simulink model "Quadrotor_Inner_Loop"  (Simulink 7.6)
settings: Solver=FixedStepDiscrete  StartTime=0.0  StopTime=10.0  FixedStep=0.01  RelTol=1e-3
libraries: passive_control x1
CloseFcn:
  | rtwprivate ssgencode ModelCloseRequest Quadrotor_Inner_Loop
settings Model: Creator=jporter  LastModifiedBy=Administrator
settings DataIOCC: LimitDataPoints=off  SaveOutput=off  SignalLogging=off  DSMLogging=off  SaveTime=off
settings OptimizationCC: InlineParams=on  EnhancedBackFolding=on  PassReuseOutputArgsAs=Individual arguments  OptimizeModelRefInitCode=on
settings HardwareCC: ProdLargestAtomicInteger=Long  ProdLargestAtomicFloat=Float  ProdIntDivRoundTo=Floor  ProdEndianess=LittleEndian  ProdHWDeviceType=ARM Compatible->ARM 7  TargetLargestAtomicInteger=Long  TargetLargestAtomicFloat=Float  TargetIntDivRoundTo=Floor  TargetEndianess=LittleEndian  TargetHWDeviceType=ARM Compatible->ARM 7
settings RTWCC: SystemTargetFile=ert.tlc  GenCodeOnly=on  TemplateMakefile=ert_default_tmf  Description=Real-Time Workshop Embedded Coder  GenerateReport=on  ProcessScript=ert_make_rtw_hook  IncludeHyperlinkInReport=on  LaunchReport=on  GenerateTraceReportSl=on  GenerateTraceReportEml=on  RTWCompilerOptimization=On  CheckMdlBeforeBuild=Warning
settings CodeAppCC: IgnoreCustomStorageClasses=off
settings ERTTargetCC: MultiwordLength=2048  GenerateSampleERTMain=on  CombineSignalStateStructs=on  MultiInstanceERTCode=on  SupportComplex=off  MultiInstanceErrorCode=Warning  ERTCustomFileTemplate=example_file_process.tlc

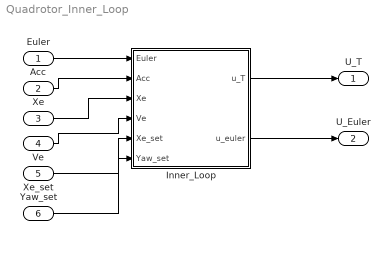
== system Quadrotor_Inner_Loop ==
  Euler : Inport  OutDataTypeStr=single  PortDimensions=[3]
  Acc : Inport  Port=2  OutDataTypeStr=single  PortDimensions=[3]
  Xe : Inport  Port=3  OutDataTypeStr=single  PortDimensions=[3]
  Ve : Inport  Port=4  OutDataTypeStr=single  PortDimensions=[3]
  Xe_set : Inport  Port=5  OutDataTypeStr=single  PortDimensions=[3]
  Yaw_set : Inport  Port=6  OutDataTypeStr=single  PortDimensions=[1]
  Inner_Loop : Subsystem
  U_T : Outport
  U_Euler : Outport  Port=2
  wires:
  Euler/1 -> Inner_Loop/1(Euler)
  Acc/1 -> Inner_Loop/2(Acc)
  Xe/1 -> Inner_Loop/3(Xe)
  Inner_Loop/1(u_T) -> U_T/1
  Inner_Loop/2(u_euler) -> U_Euler/1
  Ve/1 -> Inner_Loop/4(Ve)
  Xe_set/1 -> Inner_Loop/5(Xe_set)
  Yaw_set/1 -> Inner_Loop/6(Yaw_set)

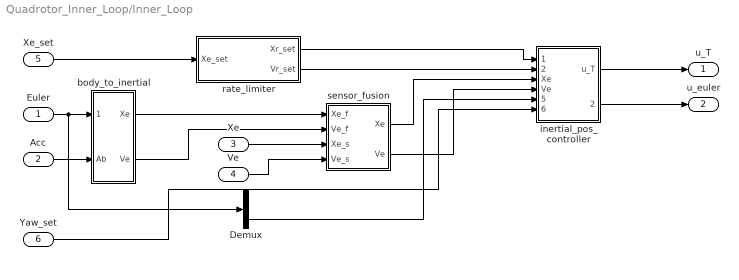
== system Quadrotor_Inner_Loop/Inner_Loop ==
  Euler : Inport  OutDataTypeStr=single  PortDimensions=[3]
  Acc : Inport  Port=2  OutDataTypeStr=single  PortDimensions=[3]
  Xe : Inport  Port=3  OutDataTypeStr=single  PortDimensions=[3]
  Ve : Inport  Port=4  OutDataTypeStr=single  PortDimensions=[3]
  Xe_set : Inport  Port=5  OutDataTypeStr=single  PortDimensions=[3]
  Yaw_set : Inport  Port=6  OutDataTypeStr=single  PortDimensions=[1]
  Demux : Demux  Outputs=3
  body_to_inertial : Subsystem
  inertial_pos_controller : Subsystem
  rate_limiter : Subsystem  mask{wn=2*pi, zeta=0.9, Vmax=2, Ts=0.01}
      mask prompts: wn "omega_n"; Vmax "Max velocity"; Ts "Sample time"
      mask init:
      | Hs_v=tf([2*zeta*wn],[1,2*zeta*wn]);
      | Hz_v=ipesh_transform(Hs_v,Ts);
      | Hs_i=tf([1],[1,0]);
      | Hz_i=ipesh_transform(Hs_i,Ts);
  sensor_fusion : Subsystem  mask{tau=.1, Ts=.01, Ts_gps=.1}
      mask prompts: tau "low-pass time constant (sec) [tau]"; Ts "Sample time [Ts]"; Ts_gps "GPS Sample Time [Ts_gps]"
  u_T : Outport  OutDataTypeStr=single  PortDimensions=[1]
  u_euler : Outport  Port=2  OutDataTypeStr=single  PortDimensions=[3]
  wires:
  Xe_set/1 -> rate_limiter/1(Xe_set)
  inertial_pos_controller/2(u_euler) -> u_euler/1
  Euler/1 -> body_to_inertial/1(euler), Demux/1
  Acc/1 -> body_to_inertial/2(Ab)
  sensor_fusion/1(Xe) -> inertial_pos_controller/3(Xe)
  sensor_fusion/2(Ve) -> inertial_pos_controller/4(Ve)
  body_to_inertial/1(Xe) -> sensor_fusion/1(Xe_f)
  body_to_inertial/2(Ve) -> sensor_fusion/2(Ve_f)
  Xe/1 -> sensor_fusion/3(Xe_s)
  Ve/1 -> sensor_fusion/4(Ve_s)
  rate_limiter/1(Xr_set) -> inertial_pos_controller/1(Xe_set)
  Demux/3 -> inertial_pos_controller/5(Yaw_actual)
  Yaw_set/1 -> inertial_pos_controller/6(Yaw_set)
  rate_limiter/2(Vr_set) -> inertial_pos_controller/2(Ve_set)
  inertial_pos_controller/1(u_T) -> u_T/1

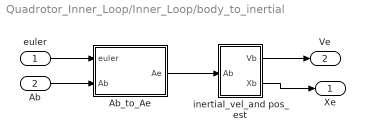
== system Quadrotor_Inner_Loop/Inner_Loop/body_to_inertial ==
  euler : Inport
  Ab : Inport  Port=2
  Ab_to_Ae : Stateflow chart  TreatAsAtomicUnit=on
  inertial_vel_and pos_est : Subsystem  mask{Ts=.01}
      mask prompts: Ts "Sample Time [Ts] (seconds):"
  Xe : Outport
  Ve : Outport  Port=2
  wires:
  euler/1 -> Ab_to_Ae/1(euler)
  Ab/1 -> Ab_to_Ae/2(Ab)
  Ab_to_Ae/1(Ae) -> inertial_vel_and pos_est/1(Ab)
  inertial_vel_and pos_est/1(Vb) -> Ve/1
  inertial_vel_and pos_est/2(Xb) -> Xe/1

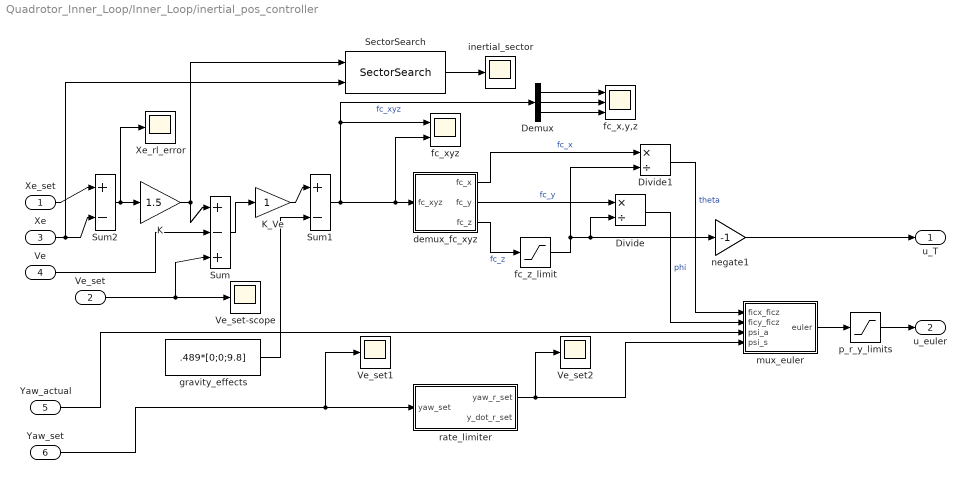
== system Quadrotor_Inner_Loop/Inner_Loop/inertial_pos_controller ==
  Xe_set : Inport
  Ve_set : Inport  Port=2
  Xe : Inport  Port=3
  Ve : Inport  Port=4
  Yaw_actual : Inport  Port=5
  Yaw_set : Inport  Port=6
  Demux : Demux  Outputs=3
  Divide : Product  Inputs=*/  OutDataTypeStr=single
  Divide1 : Product  Inputs=*/  OutDataTypeStr=single
  K : Gain  Gain=1.5  OutDataTypeStr=single
  K_Ve : Gain  ParamDataTypeStr=single  OutDataTypeStr=single
  SectorSearch : passive_control/SectorSearch  SystemSampleTime=-1
  Sum : Sum  Inputs=|+-+  AccumDataTypeStr=single  OutDataTypeStr=single
  Sum1 : Sum  Inputs=|+-  AccumDataTypeStr=single  OutDataTypeStr=single
  Sum2 : Sum  Inputs=|+-  AccumDataTypeStr=single  OutDataTypeStr=single
  Ve_set-scope : Scope
      settings: TimeRange=60  YMin=-2  YMax=2  SaveName=ScopeData2  Decimation=10
  Ve_set1 : Scope
      settings: TimeRange=60  YMin=-1  YMax=1  SaveName=ScopeData10  Decimation=10
  Ve_set2 : Scope
      settings: TimeRange=60  YMin=-1  YMax=1  SaveName=ScopeData11  Decimation=10
  Xe_rl_error : Scope
      settings: TimeRange=80  YMin=-1  YMax=1  SaveName=inertial_sector_data1  MaxDataPoints=50000
  demux_fc_xyz : Stateflow chart  TreatAsAtomicUnit=on
  fc_x,y,z : Scope  NumInputPorts=3
      settings: TimeRange=80  YMin=-1~-5~-5  YMax=1~5~5  SaveName=inertial_sector_data3  MaxDataPoints=50000
  fc_xyz : Scope  NumInputPorts=2
      settings: TimeRange=80  YMin=-1~-5  YMax=1~5  SaveName=inertial_sector_data2  MaxDataPoints=50000
  fc_z_limit : Saturate  UpperLimit=-(1/8)*3.7  LowerLimit=-4*3.7  OutDataTypeStr=single
  gravity_effects : Constant  Value=.489*[0;0;9.8]  OutDataTypeStr=single  SampleTime=.01
  inertial_sector : Scope
      settings: TimeRange=80  YMin=-1  YMax=1  SaveName=inertial_sector_data  MaxDataPoints=50000
  mux_euler : Stateflow chart  TreatAsAtomicUnit=on
  negate1 : Gain  Gain=-1  OutDataTypeStr=single
  p_r_y_limits : Saturate  UpperLimit=[pi/4,pi/4,inf]  LowerLimit=-[pi/4,pi/4,inf]  OutDataTypeStr=single
  rate_limiter : Subsystem  mask{wn=1, zeta=0.9, Vmax=2, Ts=0.01}
      mask prompts: wn "omega_n"; Vmax "Max velocity"; Ts "Sample time"
      mask init:
      | Hs_v=tf([2*zeta*wn],[1,2*zeta*wn]);
      | Hz_v=ipesh_transform(Hs_v,Ts);
      | Hs_i=tf([1],[1,0]);
      | Hz_i=ipesh_transform(Hs_i,Ts);
  u_T : Outport
  u_euler : Outport  Port=2
  wires:
  fc_z_limit/1 -> Divide1/2, Divide/2, negate1/1
  Xe_set/1 -> Sum2/1
  negate1/1 -> u_T/1
  p_r_y_limits/1 -> u_euler/1
  demux_fc_xyz/1(fc_x) -> Divide1/1  "fc_x"
  demux_fc_xyz/3(fc_z) -> fc_z_limit/1  "fc_z"
  mux_euler/1(euler) -> p_r_y_limits/1
  gravity_effects/1 -> Sum1/2
  Sum/1 -> K_Ve/1
  Xe/1 -> Sum2/2, SectorSearch/2
  Sum2/1 -> K/1, Xe_rl_error/1
  demux_fc_xyz/2(fc_y) -> Divide/1  "fc_y"
  K_Ve/1 -> Sum1/1
  Ve/1 -> Sum/2
  Divide1/1 -> mux_euler/1(ficx_ficz)  "theta"
  Divide/1 -> mux_euler/2(ficy_ficz)  "phi"
  Yaw_set/1 -> Ve_set1/1, rate_limiter/1(yaw_set)
  Yaw_actual/1 -> mux_euler/3(psi_a)
  SectorSearch/1 -> inertial_sector/1
  K/1 -> Sum/1, SectorSearch/1
  Ve_set/1 -> Sum/3, Ve_set-scope/1
  Sum1/1 -> fc_xyz/1, Demux/1, demux_fc_xyz/1(fc_xyz), fc_xyz/2  "fc_xyz"
  rate_limiter/1(yaw_r_set) -> mux_euler/4(psi_s), Ve_set2/1
  Demux/1 -> fc_x,y,z/1
  Demux/2 -> fc_x,y,z/2
  Demux/3 -> fc_x,y,z/3

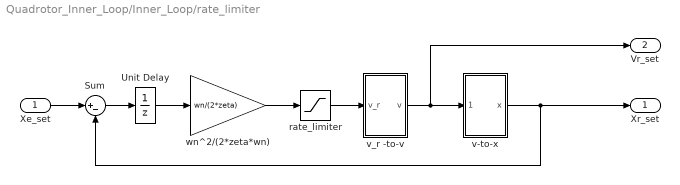
== system Quadrotor_Inner_Loop/Inner_Loop/rate_limiter ==
  Xe_set : Inport
  Sum : Sum  Inputs=|+-
  Unit Delay : UnitDelay  SampleTime=-1
  rate_limiter : Saturate  UpperLimit=Vmax*[1,1,1]  LowerLimit=-Vmax*[1,1,1]
  v-to-x : Subsystem
  v_r -to-v : Subsystem
  wn^2/(2*zeta*wn) : Gain  Gain=wn/(2*zeta)
  Xr_set : Outport
  Vr_set : Outport  Port=2
  wires:
  v_r -to-v/1(v) -> v-to-x/1(x_dot), Vr_set/1
  v-to-x/1(x) -> Sum/2, Xr_set/1
  rate_limiter/1 -> v_r -to-v/1(v_r)
  Xe_set/1 -> Sum/1
  Sum/1 -> Unit Delay/1
  wn^2/(2*zeta*wn)/1 -> rate_limiter/1
  Unit Delay/1 -> wn^2/(2*zeta*wn)/1

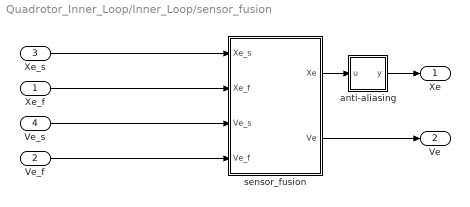
== system Quadrotor_Inner_Loop/Inner_Loop/sensor_fusion ==
  Xe_f : Inport
  Ve_f : Inport  Port=2
  Xe_s : Inport  Port=3
  Ve_s : Inport  Port=4
  anti-aliasing : Subsystem  mask{tau=tau, Ts=Ts}
      mask prompts: tau "tau (sec)"; Ts "Ts (sec)"
      mask init:
      | Hs = tf(1,[tau,1]);
      | Hz = ipesh_transform(Hs,Ts);
  sensor_fusion : Stateflow chart  TreatAsAtomicUnit=on
  Xe : Outport
  Ve : Outport  Port=2
  wires:
  Xe_f/1 -> sensor_fusion/2(Xe_f)
  Ve_f/1 -> sensor_fusion/4(Ve_f)
  sensor_fusion/1(Xe) -> anti-aliasing/1(u)
  anti-aliasing/1(y) -> Xe/1
  Xe_s/1 -> sensor_fusion/1(Xe_s)
  sensor_fusion/2(Ve) -> Ve/1
  Ve_s/1 -> sensor_fusion/3(Ve_s)

== system Quadrotor_Inner_Loop/Inner_Loop/body_to_inertial/inertial_vel_and pos_est ==
  Ab : Inport
  DT_integrator : Subsystem
  DT_integrator1 : Subsystem
  Vb : Outport
  Xb : Outport  Port=2
  wires:
  DT_integrator1/1(Xb) -> Xb/1
  Ab/1 -> DT_integrator/1(Ab)
  DT_integrator/1(Vb) -> Vb/1, DT_integrator1/1(Vb)

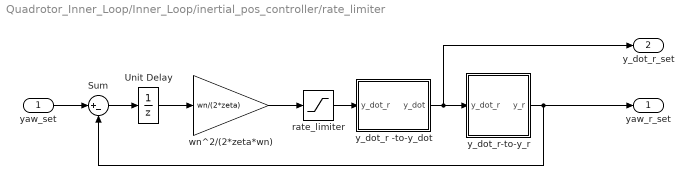
== system Quadrotor_Inner_Loop/Inner_Loop/inertial_pos_controller/rate_limiter ==
  yaw_set : Inport
  Sum : Sum  Inputs=|+-
  Unit Delay : UnitDelay  SampleTime=-1
  rate_limiter : Saturate  UpperLimit=Vmax  LowerLimit=-Vmax
  wn^2/(2*zeta*wn) : Gain  Gain=wn/(2*zeta)
  y_dot_r -to-y_dot : Subsystem
  y_dot_r-to-y_r : Subsystem
  yaw_r_set : Outport
  y_dot_r_set : Outport  Port=2
  wires:
  Unit Delay/1 -> wn^2/(2*zeta*wn)/1
  wn^2/(2*zeta*wn)/1 -> rate_limiter/1
  Sum/1 -> Unit Delay/1
  yaw_set/1 -> Sum/1
  rate_limiter/1 -> y_dot_r -to-y_dot/1(y_dot_r)
  y_dot_r-to-y_r/1(y_r) -> yaw_r_set/1, Sum/2
  y_dot_r -to-y_dot/1(y_dot) -> y_dot_r_set/1, y_dot_r-to-y_r/1(y_dot_r)

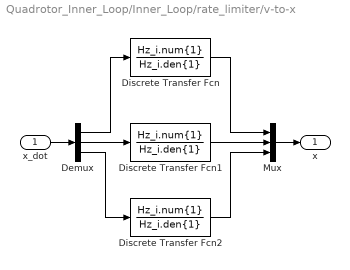
== system Quadrotor_Inner_Loop/Inner_Loop/rate_limiter/v-to-x ==
  x_dot : Inport
  Demux : Demux  Outputs=3
  Discrete Transfer Fcn : DiscreteTransferFcn  Numerator=Hz_i.num{1}  Denominator=Hz_i.den{1}  SampleTime=-1
  Discrete Transfer Fcn1 : DiscreteTransferFcn  Numerator=Hz_i.num{1}  Denominator=Hz_i.den{1}  SampleTime=-1
  Discrete Transfer Fcn2 : DiscreteTransferFcn  Numerator=Hz_i.num{1}  Denominator=Hz_i.den{1}  SampleTime=-1
  Mux : Mux  Inputs=3
  x : Outport
  wires:
  Mux/1 -> x/1
  x_dot/1 -> Demux/1
  Discrete Transfer Fcn2/1 -> Mux/3
  Demux/3 -> Discrete Transfer Fcn2/1
  Discrete Transfer Fcn1/1 -> Mux/2
  Demux/2 -> Discrete Transfer Fcn1/1
  Discrete Transfer Fcn/1 -> Mux/1
  Demux/1 -> Discrete Transfer Fcn/1

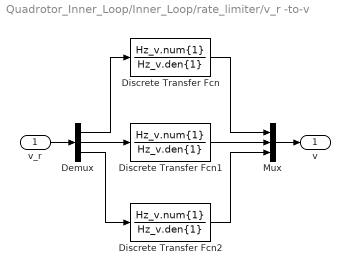
== system Quadrotor_Inner_Loop/Inner_Loop/rate_limiter/v_r -to-v ==
  v_r : Inport
  Demux : Demux  Outputs=3
  Discrete Transfer Fcn : DiscreteTransferFcn  Numerator=Hz_v.num{1}  Denominator=Hz_v.den{1}  SampleTime=-1
  Discrete Transfer Fcn1 : DiscreteTransferFcn  Numerator=Hz_v.num{1}  Denominator=Hz_v.den{1}  SampleTime=-1
  Discrete Transfer Fcn2 : DiscreteTransferFcn  Numerator=Hz_v.num{1}  Denominator=Hz_v.den{1}  SampleTime=-1
  Mux : Mux  Inputs=3
  v : Outport
  wires:
  Demux/1 -> Discrete Transfer Fcn/1
  Discrete Transfer Fcn/1 -> Mux/1
  Demux/2 -> Discrete Transfer Fcn1/1
  Discrete Transfer Fcn1/1 -> Mux/2
  Demux/3 -> Discrete Transfer Fcn2/1
  Discrete Transfer Fcn2/1 -> Mux/3
  v_r/1 -> Demux/1
  Mux/1 -> v/1

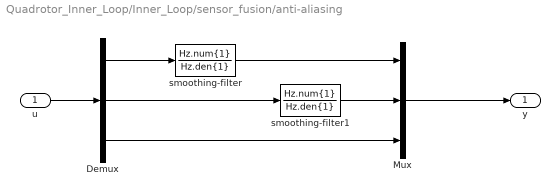
== system Quadrotor_Inner_Loop/Inner_Loop/sensor_fusion/anti-aliasing ==
  u : Inport
  Demux : Demux  Outputs=3
  Mux : Mux  Inputs=3
  smoothing-filter : DiscreteTransferFcn  Numerator=Hz.num{1}  Denominator=Hz.den{1}  SampleTime=-1
  smoothing-filter1 : DiscreteTransferFcn  Numerator=Hz.num{1}  Denominator=Hz.den{1}  SampleTime=-1
  y : Outport
  wires:
  Demux/3 -> Mux/3
  Demux/2 -> smoothing-filter1/1
  smoothing-filter1/1 -> Mux/2
  smoothing-filter/1 -> Mux/1
  Demux/1 -> smoothing-filter/1
  Mux/1 -> y/1
  u/1 -> Demux/1

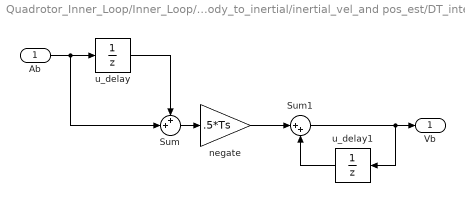
== system Quadrotor_Inner_Loop/Inner_Loop/body_to_inertial/inertial_vel_and pos_est/DT_integrator ==
  Ab : Inport
  Sum : Sum  Inputs=++|  OutDataTypeStr=single
  Sum1 : Sum  Inputs=|++  AccumDataTypeStr=single
  negate : Gain  Gain=.5*Ts  OutDataTypeStr=single
  u_delay : UnitDelay  SampleTime=-1
  u_delay1 : UnitDelay  SampleTime=-1
  Vb : Outport
  wires:
  Ab/1 -> u_delay/1, Sum/2
  u_delay/1 -> Sum/1
  Sum/1 -> negate/1
  negate/1 -> Sum1/1
  Sum1/1 -> u_delay1/1, Vb/1
  u_delay1/1 -> Sum1/2

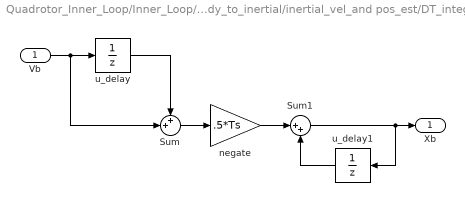
== system Quadrotor_Inner_Loop/Inner_Loop/body_to_inertial/inertial_vel_and pos_est/DT_integrator1 ==
  Vb : Inport
  Sum : Sum  Inputs=++|  OutDataTypeStr=single
  Sum1 : Sum  Inputs=|++  OutDataTypeStr=single
  negate : Gain  Gain=.5*Ts  OutDataTypeStr=single
  u_delay : UnitDelay  SampleTime=-1
  u_delay1 : UnitDelay  SampleTime=-1
  Xb : Outport  OutDataTypeStr=single  PortDimensions=[3]
  wires:
  u_delay1/1 -> Sum1/2
  Sum1/1 -> Xb/1, u_delay1/1
  negate/1 -> Sum1/1
  Sum/1 -> negate/1
  u_delay/1 -> Sum/1
  Vb/1 -> Sum/2, u_delay/1

== system Quadrotor_Inner_Loop/Inner_Loop/inertial_pos_controller/rate_limiter/y_dot_r -to-y_dot ==
  y_dot_r : Inport
  Discrete Transfer Fcn : DiscreteTransferFcn  Numerator=Hz_v.num{1}  Denominator=Hz_v.den{1}  SampleTime=-1
  y_dot : Outport
  wires:
  Discrete Transfer Fcn/1 -> y_dot/1
  y_dot_r/1 -> Discrete Transfer Fcn/1

== system Quadrotor_Inner_Loop/Inner_Loop/inertial_pos_controller/rate_limiter/y_dot_r-to-y_r ==
  y_dot_r : Inport
  Discrete Transfer Fcn : DiscreteTransferFcn  Numerator=Hz_i.num{1}  Denominator=Hz_i.den{1}  SampleTime=-1
  y_r : Outport
  wires:
  y_dot_r/1 -> Discrete Transfer Fcn/1
  Discrete Transfer Fcn/1 -> y_r/1

== matlab function Inner_Loop/body_to_inertial/Ab_to_Ae ==
  data: euler input single size=[3]; Ae output single size=[3]; Ab input single size=[3]
function Ae = fcn(euler, Ab)
% This block supports the Embedded MATLAB subset.
% See the help menu for details. 
phi=euler(1);
theta=euler(2);
psi=euler(3);
c_phi=cos(phi);
c_theta=cos(theta);
c_psi=cos(psi);
s_phi=sin(phi);
s_theta=sin(theta);
s_psi=sin(psi);
R=single([c_theta*c_psi, c_theta*s_psi, -s_theta;
   s_phi*s_theta*c_psi-c_phi*s_psi, s_phi*s_theta*s_psi+c_phi*c_psi, c_theta*s_phi;
   c_phi*s_theta*c_psi+s_phi*s_psi, c_phi*s_theta*s_psi-s_phi*c_psi, c_theta*c_phi]);
%R=single(zeros(3,3));
%R(1,1)=c_theta*c_psi;
%R(1,2)=c_theta*s_psi;
%R(1,3)=-s_theta;
%R(2,1)=s_phi*s_theta*c_psi - c_phi*s_psi;
%R(2,2)=s_phi*s_theta*s_psi + c_phi*c_psi;
%R(2,3)=c_theta*s_phi;
%R(3,1)=c_phi*s_theta*c_psi + s_phi*s_psi;
%R(3,2)=c_phi*s_theta*s_psi - s_phi*c_psi;
%R(3,3)=c_theta*c_phi;
Ae= transpose(R) * Ab;
%Ae= single(Aed);

== matlab function Inner_Loop/inertial_pos_controller/demux_fc_xyz ==
  data: fc_xyz input single size=[3]; fc_x output single size=[1]; fc_y output single size=[1]; fc_z output single size=[1]
function [fc_x,fc_y, fc_z] = fcn(fc_xyz)
% This block supports the Embedded MATLAB subset.
% See the help menu for details. 
fc_x=fc_xyz(1);
fc_y=fc_xyz(2);
fc_z=fc_xyz(3);

== matlab function Inner_Loop/inertial_pos_controller/mux_euler ==
  data: ficx_ficz input single size=[1]; euler output single size=[3]; ficy_ficz input single size=[1]; psi_a input single size=[1]; psi_s input single
function euler = fcn(ficx_ficz, ficy_ficz, psi_a, psi_s)
% This block supports the Embedded MATLAB subset.
% See the help menu for details. 

A = [sin(psi_a) -cos(psi_a); cos(psi_a) sin(psi_a)];
% Get [phi, theta] 
euler_angs = (A * [ficx_ficz; ficy_ficz])';

euler=[euler_angs(1);euler_angs(2);psi_s];

== matlab function Inner_Loop/sensor_fusion/sensor_fusion ==
  data: Xe_s input double; Xe output double; Xe_f input double; Ve_s input double; Ve_f input double; Ve output double; Ts_gps parameter double; Ts parameter double
function [Xe,Ve] = fcn(Xe_s, Xe_f, Ve_s, Ve_f, Ts_gps, Ts)
%Fuse the gps measurements Xe_s and Ve_s with the
%faster inertial sensor measurements Xe_f, Ve_f
%N.B. the height is updated by a fast pressure sensor so we always
%pass through the z-component of Xe_s and Ve_s
persistent count;
persistent dXe_s_last;
persistent dVe_s_last;
persistent dXe_s_last_2;
if isempty(count)
    count = floor(Ts_gps/Ts);
    dXe_s_last = Xe_s-Xe_f;
    dXe_s_last_2 = dXe_s_last;
    dVe_s_last = Ve_s-Ve_f;
    dXe_s_last(3)=0;
    dVe_s_last(3)=0;
end
if count == floor(Ts_gps/Ts)
    count = 1; 
    temp = ((Xe_s(1:2)-Xe_f(1:2)) + dXe_s_last(1:2) + dXe_s_last_2(1:2))/3;
    dXe_s_last_2 = dXe_s_last;
    dXe_s_last(1:2) = temp;
    dVe_s_last(1:2) = Ve_s(1:2)-Ve_f(1:2);
else
    count = count + 1;
end
Xe = Xe_f + dXe_s_last;
Ve = Ve_f + dVe_s_last;
Xe(3) = Xe_s(3);
Ve(3) = Ve_s(3);
